simulink model "baseModel"  (R2016b)
settings: Solver=ode14x  StartTime=0.0  StopTime=20  FixedStep=0.01  RelTol=1e-3
values from neighbouring files (symbols this model uses):
  b = (Km*Kb/R)*((2*pi/60))^2    (= 2.64985465309e-07)    [params.m]
  encRes = 64    [params.m]
  gearRatio = 4096/27    (= 151.703703704)    [params.m]
  geom_factor = (0.160 + 0.146)/2    (= 0.153)    [params.m]
  J = 2.7*(10^(-7))    (= 2.7e-07)    [params.m]
  Kb = 0.00152/(2*pi/60)    (= 0.01451493081)    [params.m]
  Km = 0.0145    [params.m]
  L = 0.0002    [params.m]
  pwmRes = 4096    [params.m]
  R = 8.71    [params.m]
  supplyVoltage = 12    [params.m]
  wheelRadius = 0.03    [params.m]
libraries: simulink x7
settings Model: Creator=Mundt  LastModifiedBy=Mundt

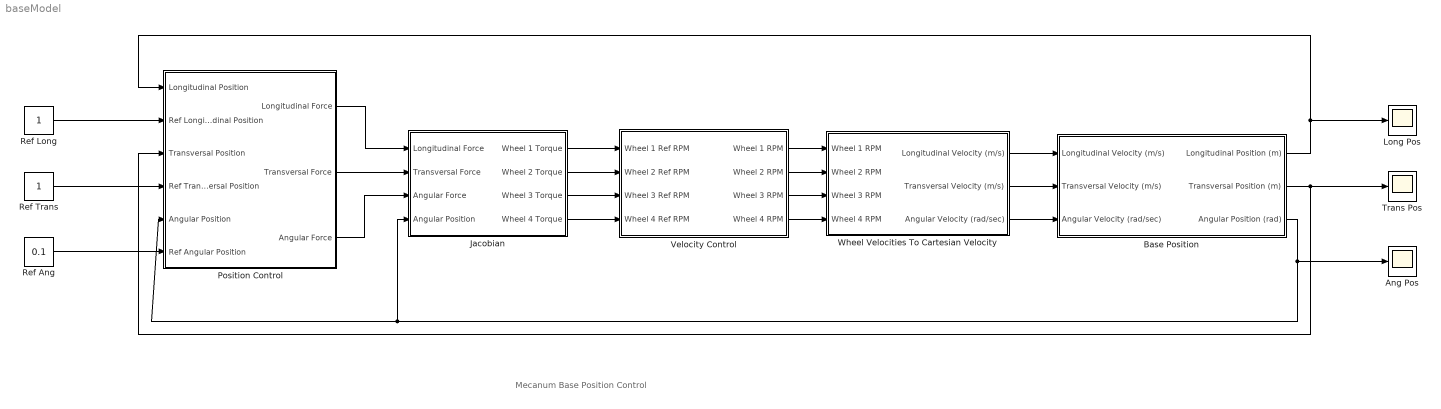
== system baseModel ==
  note: Mecanum Base Position Control
  Ang Pos : Scope
  Base Position : Subsystem
  Jacobian : Subsystem
  Long Pos : Scope
  Position Control : Subsystem
  Ref Ang : Constant  Value=0.1
  Ref Long : Constant
  Ref Trans : Constant
  Trans Pos : Scope
  Velocity Control : Subsystem
  Wheel Velocities To Cartesian Velocity : Subsystem
  wires:
  Velocity Control/1(Wheel 1 RPM) -> Wheel Velocities To Cartesian Velocity/1(Wheel 1 RPM)
  Velocity Control/2(Wheel 2 RPM) -> Wheel Velocities To Cartesian Velocity/2(Wheel 2 RPM)
  Velocity Control/3(Wheel 3 RPM) -> Wheel Velocities To Cartesian Velocity/3(Wheel 3 RPM)
  Velocity Control/4(Wheel 4 RPM) -> Wheel Velocities To Cartesian Velocity/4(Wheel 4 RPM)
  Jacobian/1(Wheel 1 Torque) -> Velocity Control/1(Wheel 1 Ref RPM)
  Jacobian/2(Wheel 2 Torque) -> Velocity Control/2(Wheel 2 Ref RPM)
  Jacobian/3(Wheel 3 Torque) -> Velocity Control/3(Wheel 3 Ref RPM)
  Jacobian/4(Wheel 4 Torque) -> Velocity Control/4(Wheel 4 Ref RPM)
  Wheel Velocities To Cartesian Velocity/1(Longitudinal Velocity (m/s)) -> Base Position/1(Longitudinal Velocity (m/s))
  Wheel Velocities To Cartesian Velocity/2(Transversal Velocity (m/s)) -> Base Position/2(Transversal Velocity (m/s))
  Wheel Velocities To Cartesian Velocity/3(Angular Velocity (rad/sec)) -> Base Position/3(Angular Velocity (rad/sec))
  Base Position/3(Angular Position (rad)) -> Ang Pos/1, Position Control/5(Angular Position), Jacobian/4(Angular Position)
  Position Control/1(Longitudinal Force) -> Jacobian/1(Longitudinal Force)
  Position Control/2(Transversal Force) -> Jacobian/2(Transversal Force)
  Position Control/3(Angular Force) -> Jacobian/3(Angular Force)
  Base Position/1(Longitudinal Position (m)) -> Long Pos/1, Position Control/1(Longitudinal Position)
  Ref Long/1 -> Position Control/2(Ref Longitudinal Position)
  Base Position/2(Transversal Position (m)) -> Trans Pos/1, Position Control/3(Transversal Position)
  Ref Trans/1 -> Position Control/4(Ref Transversal Position)
  Ref Ang/1 -> Position Control/6(Ref Angular Position)

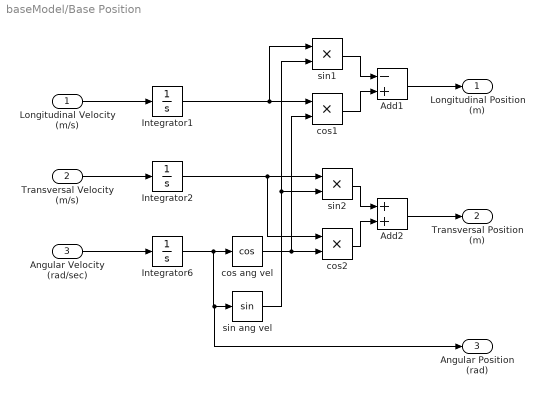
== system baseModel/Base Position ==
  Longitudinal Velocity (m/s) : Inport
  Transversal Velocity (m/s) : Inport  Port=2
  Angular Velocity (rad/sec) : Inport  Port=3
  Add1 : Sum  Inputs=-+
  Add2 : Sum
  Integrator1 : Integrator
  Integrator2 : Integrator
  Integrator6 : Integrator
  cos ang vel : Trigonometry  Operator=cos
  cos1 : Product
  cos2 : Product
  sin ang vel : Trigonometry
  sin1 : Product
  sin2 : Product
  Longitudinal Position (m) : Outport
  Transversal Position (m) : Outport  Port=2
  Angular Position (rad) : Outport  Port=3
  wires:
  Angular Velocity (rad/sec)/1 -> Integrator6/1
  Longitudinal Velocity (m/s)/1 -> Integrator1/1
  Transversal Velocity (m/s)/1 -> Integrator2/1
  Integrator6/1 -> Angular Position (rad)/1, sin ang vel/1, cos ang vel/1
  Integrator2/1 -> cos2/1, sin2/1
  Integrator1/1 -> sin1/1, cos1/1
  cos ang vel/1 -> cos1/2, cos2/2
  sin ang vel/1 -> sin2/2, sin1/2
  cos1/1 -> Add1/2
  sin1/1 -> Add1/1
  Add1/1 -> Longitudinal Position (m)/1
  sin2/1 -> Add2/1
  cos2/1 -> Add2/2
  Add2/1 -> Transversal Position (m)/1

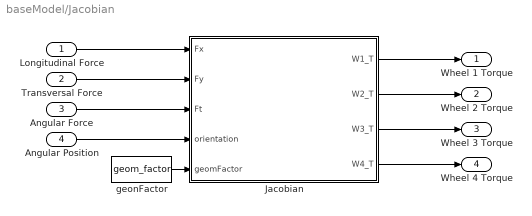
== system baseModel/Jacobian ==
  Longitudinal Force : Inport
  Transversal Force : Inport  Port=2
  Angular Force : Inport  Port=3
  Angular Position : Inport  Port=4
  Jacobian : MATLAB Function  TreatAsAtomicUnit=on
  geonFactor : Constant  Value=geom_factor
  Wheel 1 Torque : Outport
  Wheel 2 Torque : Outport  Port=2
  Wheel 3 Torque : Outport  Port=3
  Wheel 4 Torque : Outport  Port=4
  wires:
  Jacobian/2(W2_T) -> Wheel 2 Torque/1
  Jacobian/1(W1_T) -> Wheel 1 Torque/1
  Jacobian/3(W3_T) -> Wheel 3 Torque/1
  Jacobian/4(W4_T) -> Wheel 4 Torque/1
  Transversal Force/1 -> Jacobian/2(Fy)
  Angular Force/1 -> Jacobian/3(Ft)
  Angular Position/1 -> Jacobian/4(orientation)
  Longitudinal Force/1 -> Jacobian/1(Fx)
  geonFactor/1 -> Jacobian/5(geomFactor)

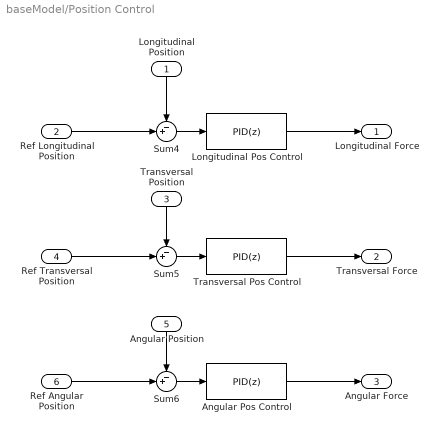
== system baseModel/Position Control ==
  Longitudinal Position : Inport
  Ref Longitudinal Position : Inport  Port=2
  Transversal Position : Inport  Port=3
  Ref Transversal Position : Inport  Port=4
  Angular Position : Inport  Port=5
  Ref Angular Position : Inport  Port=6
  Angular Pos Control : simulink/Continuous/PID Controller  Controller=PID  TimeDomain=Discrete-time  SampleTime=0.1  IntegratorMethod=Forward Euler  FilterMethod=Forward Euler  Form=Parallel  UseFilter=off  ControllerParametersSource=internal  P=1000  I=0  D=0  N=2.61986386907553  InitialConditionSource=internal  InitialConditionForIntegrator=0  InitialConditionForFilter=0  ExternalReset=none  LimitOutput=on  UpperSaturationLimit=4096  LowerSaturationLimit=-4096  LinearizeAsGain=off  AntiWindupMode=none  Kb=1  TrackingMode=off  Kt=1  PParamMin=[]  PParamMax=[]  IParamMin=[]  IParamMax=[]  DParamMin=[]  DParamMax=[]  NParamMin=[]  NParamMax=[]  KbParamMin=[]  KbParamMax=[]  KtParamMin=[]  KtParamMax=[]  POutMin=[]  POutMax=[]  IOutMin=[]  IOutMax=[]  DOutMin=[]  DOutMax=[]  NOutMin=[]  NOutMax=[]  KbOutMin=[]  KbOutMax=[]  KtOutMin=[]  KtOutMax=[]  IntegratorOutMin=[]  IntegratorOutMax=[]  FilterOutMin=[]  FilterOutMax=[]  SumOutMin=[]  SumOutMax=[]  SumI1OutMin=[]  SumI1OutMax=[]  SumI2OutMin=[]  SumI2OutMax=[]  SumI3OutMin=[]  SumI3OutMax=[]  SumDOutMin=[]  SumDOutMax=[]  SaturationOutMin=[]  SaturationOutMax=[]  IntegratorContinuousStateAttributes=''  IntegratorStateMustResolveToSignalObject=off  IntegratorRTWStateStorageClass=Auto  FilterContinuousStateAttributes=''  FilterStateMustResolveToSignalObject=off  FilterRTWStateStorageClass=Auto  DifferentiatorICPrevScaledInput=0  DifferentiatorOutMin=[]  DifferentiatorOutMax=[]
  Longitudinal Pos Control : simulink/Continuous/PID Controller  Controller=PID  TimeDomain=Discrete-time  SampleTime=0.1  IntegratorMethod=Forward Euler  FilterMethod=Forward Euler  Form=Parallel  UseFilter=off  ControllerParametersSource=internal  P=2000  I=0  D=0  N=2.61986386907553  InitialConditionSource=internal  InitialConditionForIntegrator=0  InitialConditionForFilter=0  ExternalReset=none  LimitOutput=on  UpperSaturationLimit=4096  LowerSaturationLimit=-4096  LinearizeAsGain=off  AntiWindupMode=none  Kb=1  TrackingMode=off  Kt=1  PParamMin=[]  PParamMax=[]  IParamMin=[]  IParamMax=[]  DParamMin=[]  DParamMax=[]  NParamMin=[]  NParamMax=[]  KbParamMin=[]  KbParamMax=[]  KtParamMin=[]  KtParamMax=[]  POutMin=[]  POutMax=[]  IOutMin=[]  IOutMax=[]  DOutMin=[]  DOutMax=[]  NOutMin=[]  NOutMax=[]  KbOutMin=[]  KbOutMax=[]  KtOutMin=[]  KtOutMax=[]  IntegratorOutMin=[]  IntegratorOutMax=[]  FilterOutMin=[]  FilterOutMax=[]  SumOutMin=[]  SumOutMax=[]  SumI1OutMin=[]  SumI1OutMax=[]  SumI2OutMin=[]  SumI2OutMax=[]  SumI3OutMin=[]  SumI3OutMax=[]  SumDOutMin=[]  SumDOutMax=[]  SaturationOutMin=[]  SaturationOutMax=[]  IntegratorContinuousStateAttributes=''  IntegratorStateMustResolveToSignalObject=off  IntegratorRTWStateStorageClass=Auto  FilterContinuousStateAttributes=''  FilterStateMustResolveToSignalObject=off  FilterRTWStateStorageClass=Auto  DifferentiatorICPrevScaledInput=0  DifferentiatorOutMin=[]  DifferentiatorOutMax=[]
  Sum4 : Sum  Inputs=-+|
  Sum5 : Sum  Inputs=-+|
  Sum6 : Sum  Inputs=-+|
  Transversal Pos Control : simulink/Continuous/PID Controller  Controller=PID  TimeDomain=Discrete-time  SampleTime=0.1  IntegratorMethod=Forward Euler  FilterMethod=Forward Euler  Form=Parallel  UseFilter=off  ControllerParametersSource=internal  P=2000  I=0  D=0  N=2.61986386907553  InitialConditionSource=internal  InitialConditionForIntegrator=0  InitialConditionForFilter=0  ExternalReset=none  LimitOutput=on  UpperSaturationLimit=4096  LowerSaturationLimit=-4096  LinearizeAsGain=off  AntiWindupMode=none  Kb=1  TrackingMode=off  Kt=1  PParamMin=[]  PParamMax=[]  IParamMin=[]  IParamMax=[]  DParamMin=[]  DParamMax=[]  NParamMin=[]  NParamMax=[]  KbParamMin=[]  KbParamMax=[]  KtParamMin=[]  KtParamMax=[]  POutMin=[]  POutMax=[]  IOutMin=[]  IOutMax=[]  DOutMin=[]  DOutMax=[]  NOutMin=[]  NOutMax=[]  KbOutMin=[]  KbOutMax=[]  KtOutMin=[]  KtOutMax=[]  IntegratorOutMin=[]  IntegratorOutMax=[]  FilterOutMin=[]  FilterOutMax=[]  SumOutMin=[]  SumOutMax=[]  SumI1OutMin=[]  SumI1OutMax=[]  SumI2OutMin=[]  SumI2OutMax=[]  SumI3OutMin=[]  SumI3OutMax=[]  SumDOutMin=[]  SumDOutMax=[]  SaturationOutMin=[]  SaturationOutMax=[]  IntegratorContinuousStateAttributes=''  IntegratorStateMustResolveToSignalObject=off  IntegratorRTWStateStorageClass=Auto  FilterContinuousStateAttributes=''  FilterStateMustResolveToSignalObject=off  FilterRTWStateStorageClass=Auto  DifferentiatorICPrevScaledInput=0  DifferentiatorOutMin=[]  DifferentiatorOutMax=[]
  Longitudinal Force : Outport
  Transversal Force : Outport  Port=2
  Angular Force : Outport  Port=3
  wires:
  Angular Position/1 -> Sum6/1
  Longitudinal Position/1 -> Sum4/1
  Angular Pos Control/1 -> Angular Force/1
  Transversal Pos Control/1 -> Transversal Force/1
  Transversal Position/1 -> Sum5/1
  Sum4/1 -> Longitudinal Pos Control/1
  Ref Angular Position/1 -> Sum6/2
  Sum5/1 -> Transversal Pos Control/1
  Ref Transversal Position/1 -> Sum5/2
  Sum6/1 -> Angular Pos Control/1
  Ref Longitudinal Position/1 -> Sum4/2
  Longitudinal Pos Control/1 -> Longitudinal Force/1

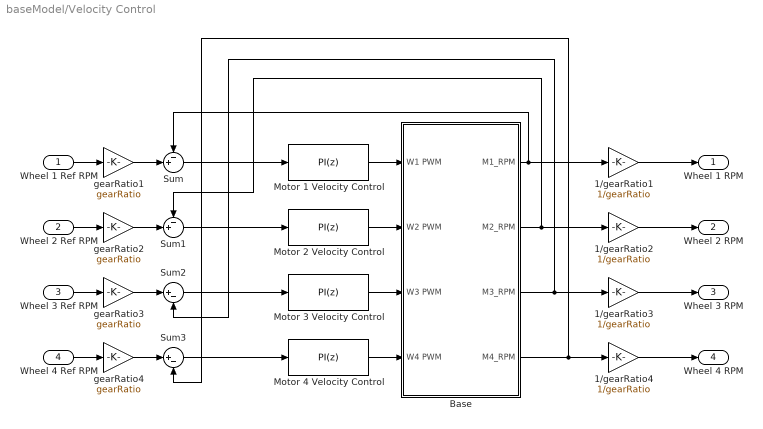
== system baseModel/Velocity Control ==
  Wheel 1 Ref RPM : Inport
  Wheel 2 Ref RPM : Inport  Port=2
  Wheel 3 Ref RPM : Inport  Port=3
  Wheel 4 Ref RPM : Inport  Port=4
  1/gearRatio{1..4} (4 alike) : Gain  Gain=1/gearRatio
  Base : Subsystem
  Motor 1 Velocity Control : simulink/Continuous/PID Controller  Controller=PI  TimeDomain=Discrete-time  SampleTime=0.01  IntegratorMethod=Forward Euler  FilterMethod=Forward Euler  Form=Parallel  UseFilter=on  ControllerParametersSource=internal  P=0.39976  I=23.7406  D=0  N=100  InitialConditionSource=internal  InitialConditionForIntegrator=0  InitialConditionForFilter=0  ExternalReset=none  LimitOutput=off  UpperSaturationLimit=inf  LowerSaturationLimit=-inf  LinearizeAsGain=off  AntiWindupMode=none  Kb=1  TrackingMode=off  Kt=1  PParamMin=[]  PParamMax=[]  IParamMin=[]  IParamMax=[]  DParamMin=[]  DParamMax=[]  NParamMin=[]  NParamMax=[]  KbParamMin=[]  KbParamMax=[]  KtParamMin=[]  KtParamMax=[]  POutMin=[]  POutMax=[]  IOutMin=[]  IOutMax=[]  DOutMin=[]  DOutMax=[]  NOutMin=[]  NOutMax=[]  KbOutMin=[]  KbOutMax=[]  KtOutMin=[]  KtOutMax=[]  IntegratorOutMin=[]  IntegratorOutMax=[]  FilterOutMin=[]  FilterOutMax=[]  SumOutMin=[]  SumOutMax=[]  SumI1OutMin=[]  SumI1OutMax=[]  SumI2OutMin=[]  SumI2OutMax=[]  SumI3OutMin=[]  SumI3OutMax=[]  SumDOutMin=[]  SumDOutMax=[]  SaturationOutMin=[]  SaturationOutMax=[]  IntegratorContinuousStateAttributes=''  IntegratorStateMustResolveToSignalObject=off  IntegratorRTWStateStorageClass=Auto  FilterContinuousStateAttributes=''  FilterStateMustResolveToSignalObject=off  FilterRTWStateStorageClass=Auto  DifferentiatorICPrevScaledInput=0  DifferentiatorOutMin=[]  DifferentiatorOutMax=[]
  Motor 2 Velocity Control : simulink/Continuous/PID Controller  Controller=PI  TimeDomain=Discrete-time  SampleTime=0.01  IntegratorMethod=Forward Euler  FilterMethod=Forward Euler  Form=Parallel  UseFilter=on  ControllerParametersSource=internal  P=0.39976  I=23.7406  D=0  N=100  InitialConditionSource=internal  InitialConditionForIntegrator=0  InitialConditionForFilter=0  ExternalReset=none  LimitOutput=off  UpperSaturationLimit=inf  LowerSaturationLimit=-inf  LinearizeAsGain=off  AntiWindupMode=none  Kb=1  TrackingMode=off  Kt=1  PParamMin=[]  PParamMax=[]  IParamMin=[]  IParamMax=[]  DParamMin=[]  DParamMax=[]  NParamMin=[]  NParamMax=[]  KbParamMin=[]  KbParamMax=[]  KtParamMin=[]  KtParamMax=[]  POutMin=[]  POutMax=[]  IOutMin=[]  IOutMax=[]  DOutMin=[]  DOutMax=[]  NOutMin=[]  NOutMax=[]  KbOutMin=[]  KbOutMax=[]  KtOutMin=[]  KtOutMax=[]  IntegratorOutMin=[]  IntegratorOutMax=[]  FilterOutMin=[]  FilterOutMax=[]  SumOutMin=[]  SumOutMax=[]  SumI1OutMin=[]  SumI1OutMax=[]  SumI2OutMin=[]  SumI2OutMax=[]  SumI3OutMin=[]  SumI3OutMax=[]  SumDOutMin=[]  SumDOutMax=[]  SaturationOutMin=[]  SaturationOutMax=[]  IntegratorContinuousStateAttributes=''  IntegratorStateMustResolveToSignalObject=off  IntegratorRTWStateStorageClass=Auto  FilterContinuousStateAttributes=''  FilterStateMustResolveToSignalObject=off  FilterRTWStateStorageClass=Auto  DifferentiatorICPrevScaledInput=0  DifferentiatorOutMin=[]  DifferentiatorOutMax=[]
  Motor 3 Velocity Control : simulink/Continuous/PID Controller  Controller=PI  TimeDomain=Discrete-time  SampleTime=0.01  IntegratorMethod=Forward Euler  FilterMethod=Forward Euler  Form=Parallel  UseFilter=on  ControllerParametersSource=internal  P=0.39976  I=23.7406  D=0  N=100  InitialConditionSource=internal  InitialConditionForIntegrator=0  InitialConditionForFilter=0  ExternalReset=none  LimitOutput=off  UpperSaturationLimit=inf  LowerSaturationLimit=-inf  LinearizeAsGain=off  AntiWindupMode=none  Kb=1  TrackingMode=off  Kt=1  PParamMin=[]  PParamMax=[]  IParamMin=[]  IParamMax=[]  DParamMin=[]  DParamMax=[]  NParamMin=[]  NParamMax=[]  KbParamMin=[]  KbParamMax=[]  KtParamMin=[]  KtParamMax=[]  POutMin=[]  POutMax=[]  IOutMin=[]  IOutMax=[]  DOutMin=[]  DOutMax=[]  NOutMin=[]  NOutMax=[]  KbOutMin=[]  KbOutMax=[]  KtOutMin=[]  KtOutMax=[]  IntegratorOutMin=[]  IntegratorOutMax=[]  FilterOutMin=[]  FilterOutMax=[]  SumOutMin=[]  SumOutMax=[]  SumI1OutMin=[]  SumI1OutMax=[]  SumI2OutMin=[]  SumI2OutMax=[]  SumI3OutMin=[]  SumI3OutMax=[]  SumDOutMin=[]  SumDOutMax=[]  SaturationOutMin=[]  SaturationOutMax=[]  IntegratorContinuousStateAttributes=''  IntegratorStateMustResolveToSignalObject=off  IntegratorRTWStateStorageClass=Auto  FilterContinuousStateAttributes=''  FilterStateMustResolveToSignalObject=off  FilterRTWStateStorageClass=Auto  DifferentiatorICPrevScaledInput=0  DifferentiatorOutMin=[]  DifferentiatorOutMax=[]
  Motor 4 Velocity Control : simulink/Continuous/PID Controller  Controller=PI  TimeDomain=Discrete-time  SampleTime=0.01  IntegratorMethod=Forward Euler  FilterMethod=Forward Euler  Form=Parallel  UseFilter=on  ControllerParametersSource=internal  P=0.39976  I=23.7406  D=0  N=100  InitialConditionSource=internal  InitialConditionForIntegrator=0  InitialConditionForFilter=0  ExternalReset=none  LimitOutput=off  UpperSaturationLimit=inf  LowerSaturationLimit=-inf  LinearizeAsGain=off  AntiWindupMode=none  Kb=1  TrackingMode=off  Kt=1  PParamMin=[]  PParamMax=[]  IParamMin=[]  IParamMax=[]  DParamMin=[]  DParamMax=[]  NParamMin=[]  NParamMax=[]  KbParamMin=[]  KbParamMax=[]  KtParamMin=[]  KtParamMax=[]  POutMin=[]  POutMax=[]  IOutMin=[]  IOutMax=[]  DOutMin=[]  DOutMax=[]  NOutMin=[]  NOutMax=[]  KbOutMin=[]  KbOutMax=[]  KtOutMin=[]  KtOutMax=[]  IntegratorOutMin=[]  IntegratorOutMax=[]  FilterOutMin=[]  FilterOutMax=[]  SumOutMin=[]  SumOutMax=[]  SumI1OutMin=[]  SumI1OutMax=[]  SumI2OutMin=[]  SumI2OutMax=[]  SumI3OutMin=[]  SumI3OutMax=[]  SumDOutMin=[]  SumDOutMax=[]  SaturationOutMin=[]  SaturationOutMax=[]  IntegratorContinuousStateAttributes=''  IntegratorStateMustResolveToSignalObject=off  IntegratorRTWStateStorageClass=Auto  FilterContinuousStateAttributes=''  FilterStateMustResolveToSignalObject=off  FilterRTWStateStorageClass=Auto  DifferentiatorICPrevScaledInput=0  DifferentiatorOutMin=[]  DifferentiatorOutMax=[]
  Sum : Sum  Inputs=-+|
  Sum1 : Sum  Inputs=-+|
  Sum2 : Sum  Inputs=|+-
  Sum3 : Sum  Inputs=|+-
  gearRatio1 : Gain  Gain=gearRatio
  gearRatio2 : Gain  Gain=gearRatio
  gearRatio3 : Gain  Gain=gearRatio
  "gearRatio4 " : Gain  Gain=gearRatio
  Wheel 1 RPM : Outport
  Wheel 2 RPM : Outport  Port=2
  Wheel 3 RPM : Outport  Port=3
  Wheel 4 RPM : Outport  Port=4
  wires:
  Wheel 4 Ref RPM/1 -> "gearRatio4 "/1
  Wheel 3 Ref RPM/1 -> gearRatio3/1
  gearRatio2/1 -> Sum1/2
  Sum/1 -> Motor 1 Velocity Control/1
  Wheel 1 Ref RPM/1 -> gearRatio1/1
  "gearRatio4 "/1 -> Sum3/1
  Wheel 2 Ref RPM/1 -> gearRatio2/1
  Base/1(M1_RPM) -> Sum/1, 1/gearRatio1/1
  Base/2(M2_RPM) -> Sum1/1, 1/gearRatio2/1
  Sum3/1 -> Motor 4 Velocity Control/1
  Base/3(M3_RPM) -> Sum2/2, 1/gearRatio3/1
  Sum1/1 -> Motor 2 Velocity Control/1
  Sum2/1 -> Motor 3 Velocity Control/1
  Base/4(M4_RPM) -> Sum3/2, 1/gearRatio4/1
  Motor 1 Velocity Control/1 -> Base/1(W1 PWM)
  Motor 2 Velocity Control/1 -> Base/2(W2 PWM)
  Motor 3 Velocity Control/1 -> Base/3(W3 PWM)
  Motor 4 Velocity Control/1 -> Base/4(W4 PWM)
  gearRatio1/1 -> Sum/2
  gearRatio3/1 -> Sum2/1
  1/gearRatio1/1 -> Wheel 1 RPM/1
  1/gearRatio2/1 -> Wheel 2 RPM/1
  1/gearRatio3/1 -> Wheel 3 RPM/1
  1/gearRatio4/1 -> Wheel 4 RPM/1

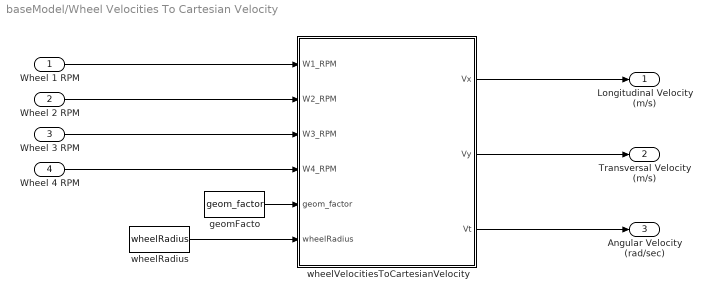
== system baseModel/Wheel Velocities To Cartesian Velocity ==
  Wheel 1 RPM : Inport
  Wheel 2 RPM : Inport  Port=2
  Wheel 3 RPM : Inport  Port=3
  Wheel 4 RPM : Inport  Port=4
  geomFacto : Constant  Value=geom_factor
  wheelRadius : Constant  Value=wheelRadius
  wheelVelocitiesToCartesianVelocity : MATLAB Function  TreatAsAtomicUnit=on
  Longitudinal Velocity (m/s) : Outport
  Transversal Velocity (m/s) : Outport  Port=2
  Angular Velocity (rad/sec) : Outport  Port=3
  wires:
  wheelRadius/1 -> wheelVelocitiesToCartesianVelocity/6(wheelRadius)
  Wheel 2 RPM/1 -> wheelVelocitiesToCartesianVelocity/2(W2_RPM)
  Wheel 4 RPM/1 -> wheelVelocitiesToCartesianVelocity/4(W4_RPM)
  geomFacto/1 -> wheelVelocitiesToCartesianVelocity/5(geom_factor)
  Wheel 1 RPM/1 -> wheelVelocitiesToCartesianVelocity/1(W1_RPM)
  Wheel 3 RPM/1 -> wheelVelocitiesToCartesianVelocity/3(W3_RPM)
  wheelVelocitiesToCartesianVelocity/3(Vt) -> Angular Velocity (rad/sec)/1
  wheelVelocitiesToCartesianVelocity/1(Vx) -> Longitudinal Velocity (m/s)/1
  wheelVelocitiesToCartesianVelocity/2(Vy) -> Transversal Velocity (m/s)/1

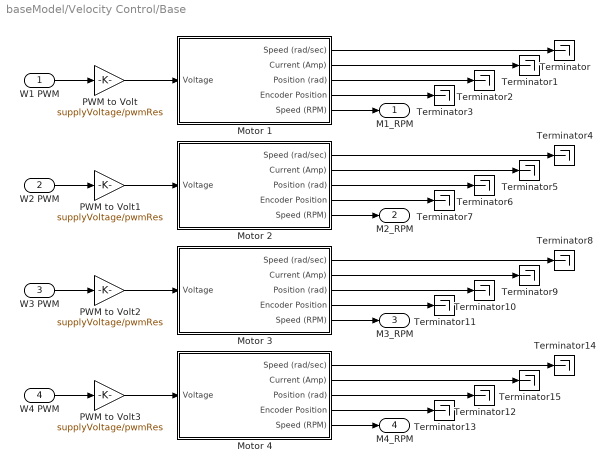
== system baseModel/Velocity Control/Base ==
  W1 PWM : Inport
  W2 PWM : Inport  Port=2
  W3 PWM : Inport  Port=3
  W4 PWM : Inport  Port=4
  Motor 1 : Subsystem
  Motor 2 : Subsystem
  Motor 3 : Subsystem
  Motor 4 : Subsystem
  PWM to Volt{,1..3} (4 alike) : Gain  Gain=supplyVoltage/pwmRes
  Terminator{,1..15} (16 alike) : Terminator
  M1_RPM : Outport
  M2_RPM : Outport  Port=2
  M3_RPM : Outport  Port=3
  M4_RPM : Outport  Port=4
  wires:
  W1 PWM/1 -> PWM to Volt/1
  PWM to Volt/1 -> Motor 1/1(Voltage)
  PWM to Volt1/1 -> Motor 2/1(Voltage)
  W2 PWM/1 -> PWM to Volt1/1
  PWM to Volt2/1 -> Motor 3/1(Voltage)
  W3 PWM/1 -> PWM to Volt2/1
  PWM to Volt3/1 -> Motor 4/1(Voltage)
  W4 PWM/1 -> PWM to Volt3/1
  Motor 1/5(Speed (RPM)) -> M1_RPM/1
  Motor 2/5(Speed (RPM)) -> M2_RPM/1
  Motor 3/5(Speed (RPM)) -> M3_RPM/1
  Motor 4/5(Speed (RPM)) -> M4_RPM/1
  Motor 1/1(Speed (rad/sec)) -> Terminator/1
  Motor 1/2(Current (Amp)) -> Terminator1/1
  Motor 1/3(Position (rad)) -> Terminator2/1
  Motor 1/4(Encoder Position) -> Terminator3/1
  Motor 2/1(Speed (rad/sec)) -> Terminator4/1
  Motor 2/2(Current (Amp)) -> Terminator5/1
  Motor 2/3(Position (rad)) -> Terminator6/1
  Motor 2/4(Encoder Position) -> Terminator7/1
  Motor 3/1(Speed (rad/sec)) -> Terminator8/1
  Motor 3/2(Current (Amp)) -> Terminator9/1
  Motor 3/3(Position (rad)) -> Terminator10/1
  Motor 3/4(Encoder Position) -> Terminator11/1
  Motor 4/1(Speed (rad/sec)) -> Terminator14/1
  Motor 4/2(Current (Amp)) -> Terminator15/1
  Motor 4/3(Position (rad)) -> Terminator12/1
  Motor 4/4(Encoder Position) -> Terminator13/1

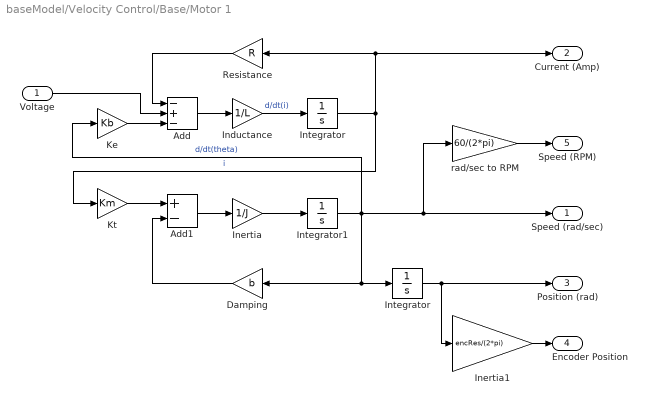
== system baseModel/Velocity Control/Base/Motor 1 ==
  Voltage : Inport
  Add : Sum  Inputs=-+-
  Add1 : Sum  Inputs=+-
  Damping : Gain  Gain=b
  Inductance : Gain  Gain=1/L
  Inertia : Gain  Gain=1/J
  Inertia1 : Gain  Gain=encRes/(2*pi)
  Integrator : Integrator
  "Integrator " : Integrator
  Integrator1 : Integrator
  Ke : Gain  Gain=Kb
  Kt : Gain  Gain=Km
  Resistance : Gain  Gain=R
  rad/sec to RPM : Gain  Gain=60/(2*pi)
  Speed (rad/sec) : Outport
  Current (Amp) : Outport  Port=2
  Position (rad) : Outport  Port=3
  Encoder Position : Outport  Port=4
  Speed (RPM) : Outport  Port=5
  wires:
  Resistance/1 -> Add/1
  Ke/1 -> Add/3
  Inertia/1 -> Integrator1/1
  Voltage/1 -> Add/2
  Damping/1 -> Add1/2
  Kt/1 -> Add1/1
  Add1/1 -> Inertia/1
  Inductance/1 -> Integrator/1  "d/dt(i)"
  Add/1 -> Inductance/1
  Integrator1/1 -> rad/sec to RPM/1, Speed (rad/sec)/1, Ke/1, "Integrator "/1, Damping/1  "d/dt(theta)"
  Integrator/1 -> Current (Amp)/1, Resistance/1, Kt/1  "i"
  "Integrator "/1 -> Inertia1/1, Position (rad)/1
  Inertia1/1 -> Encoder Position/1
  rad/sec to RPM/1 -> Speed (RPM)/1

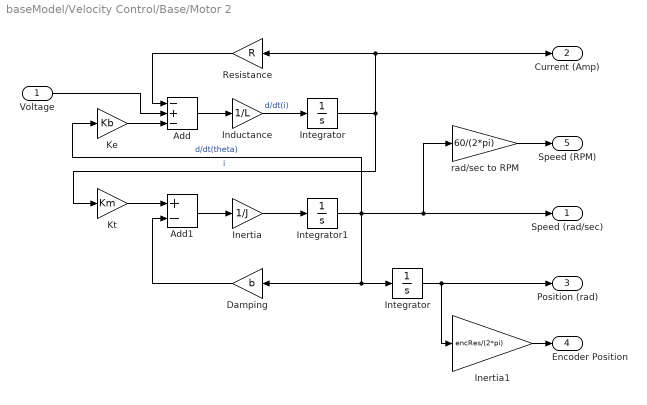
== system baseModel/Velocity Control/Base/Motor 2 ==
  Voltage : Inport
  Add : Sum  Inputs=-+-
  Add1 : Sum  Inputs=+-
  Damping : Gain  Gain=b
  Inductance : Gain  Gain=1/L
  Inertia : Gain  Gain=1/J
  Inertia1 : Gain  Gain=encRes/(2*pi)
  Integrator : Integrator
  "Integrator " : Integrator
  Integrator1 : Integrator
  Ke : Gain  Gain=Kb
  Kt : Gain  Gain=Km
  Resistance : Gain  Gain=R
  rad/sec to RPM : Gain  Gain=60/(2*pi)
  Speed (rad/sec) : Outport
  Current (Amp) : Outport  Port=2
  Position (rad) : Outport  Port=3
  Encoder Position : Outport  Port=4
  Speed (RPM) : Outport  Port=5
  wires:
  rad/sec to RPM/1 -> Speed (RPM)/1
  Inertia1/1 -> Encoder Position/1
  "Integrator "/1 -> Position (rad)/1, Inertia1/1
  Integrator/1 -> Kt/1, Resistance/1, Current (Amp)/1  "i"
  Integrator1/1 -> Damping/1, "Integrator "/1, Ke/1, Speed (rad/sec)/1, rad/sec to RPM/1  "d/dt(theta)"
  Add/1 -> Inductance/1
  Inductance/1 -> Integrator/1  "d/dt(i)"
  Add1/1 -> Inertia/1
  Kt/1 -> Add1/1
  Damping/1 -> Add1/2
  Voltage/1 -> Add/2
  Inertia/1 -> Integrator1/1
  Ke/1 -> Add/3
  Resistance/1 -> Add/1

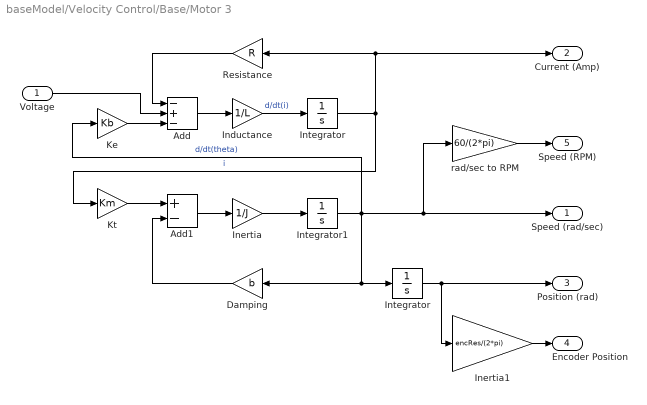
== system baseModel/Velocity Control/Base/Motor 3 ==
  Voltage : Inport
  Add : Sum  Inputs=-+-
  Add1 : Sum  Inputs=+-
  Damping : Gain  Gain=b
  Inductance : Gain  Gain=1/L
  Inertia : Gain  Gain=1/J
  Inertia1 : Gain  Gain=encRes/(2*pi)
  Integrator : Integrator
  "Integrator " : Integrator
  Integrator1 : Integrator
  Ke : Gain  Gain=Kb
  Kt : Gain  Gain=Km
  Resistance : Gain  Gain=R
  rad/sec to RPM : Gain  Gain=60/(2*pi)
  Speed (rad/sec) : Outport
  Current (Amp) : Outport  Port=2
  Position (rad) : Outport  Port=3
  Encoder Position : Outport  Port=4
  Speed (RPM) : Outport  Port=5
  wires:
  rad/sec to RPM/1 -> Speed (RPM)/1
  Inertia1/1 -> Encoder Position/1
  "Integrator "/1 -> Position (rad)/1, Inertia1/1
  Integrator/1 -> Kt/1, Resistance/1, Current (Amp)/1  "i"
  Integrator1/1 -> Damping/1, "Integrator "/1, Ke/1, Speed (rad/sec)/1, rad/sec to RPM/1  "d/dt(theta)"
  Add/1 -> Inductance/1
  Inductance/1 -> Integrator/1  "d/dt(i)"
  Add1/1 -> Inertia/1
  Kt/1 -> Add1/1
  Damping/1 -> Add1/2
  Voltage/1 -> Add/2
  Inertia/1 -> Integrator1/1
  Ke/1 -> Add/3
  Resistance/1 -> Add/1

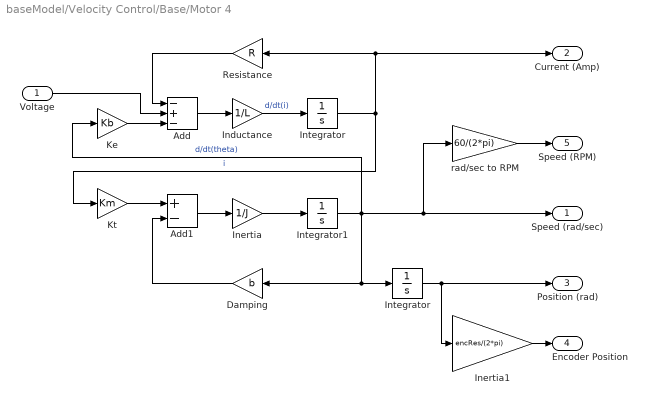
== system baseModel/Velocity Control/Base/Motor 4 ==
  Voltage : Inport
  Add : Sum  Inputs=-+-
  Add1 : Sum  Inputs=+-
  Damping : Gain  Gain=b
  Inductance : Gain  Gain=1/L
  Inertia : Gain  Gain=1/J
  Inertia1 : Gain  Gain=encRes/(2*pi)
  Integrator : Integrator
  "Integrator " : Integrator
  Integrator1 : Integrator
  Ke : Gain  Gain=Kb
  Kt : Gain  Gain=Km
  Resistance : Gain  Gain=R
  rad/sec to RPM : Gain  Gain=60/(2*pi)
  Speed (rad/sec) : Outport
  Current (Amp) : Outport  Port=2
  Position (rad) : Outport  Port=3
  Encoder Position : Outport  Port=4
  Speed (RPM) : Outport  Port=5
  wires:
  Resistance/1 -> Add/1
  Ke/1 -> Add/3
  Inertia/1 -> Integrator1/1
  Voltage/1 -> Add/2
  Damping/1 -> Add1/2
  Kt/1 -> Add1/1
  Add1/1 -> Inertia/1
  Inductance/1 -> Integrator/1  "d/dt(i)"
  Add/1 -> Inductance/1
  Integrator1/1 -> rad/sec to RPM/1, Speed (rad/sec)/1, Ke/1, "Integrator "/1, Damping/1  "d/dt(theta)"
  Integrator/1 -> Current (Amp)/1, Resistance/1, Kt/1  "i"
  "Integrator "/1 -> Inertia1/1, Position (rad)/1
  Inertia1/1 -> Encoder Position/1
  rad/sec to RPM/1 -> Speed (RPM)/1

== matlab function baseModel/Wheel Velocities To Cartesian Velocity/wheelVelocitiesToCartesianVelocity ==
  data: W1_RPM input; Vx output; W2_RPM input; W3_RPM input; W4_RPM input; Vy output; Vt output; geom_factor input; wheelRadius input
function [Vx, Vy, Vt] = fcn(W1_RPM, W2_RPM, W3_RPM, W4_RPM, geom_factor, wheelRadius )

W1_angVel = W1_RPM * 2 * pi / 60;
W2_angVel = W2_RPM * 2 * pi / 60;
W3_angVel = W3_RPM * 2 * pi / 60;
W4_angVel = W4_RPM * 2 * pi / 60;

Vx = (W1_angVel + W2_angVel + W3_angVel + W4_angVel) * wheelRadius / 4;
Vy = (W1_angVel - W2_angVel - W3_angVel + W4_angVel) * wheelRadius / 4;
Vt = (W1_angVel - W2_angVel + W3_angVel - W4_angVel) * wheelRadius /(4 * geom_factor);

== matlab function baseModel/Jacobian/Jacobian ==
  data: Fx input; W1_T output; Fy input; Ft input; orientation input; W2_T output; W3_T output; W4_T output; geomFactor input
function [W1_T, W2_T, W3_T, W4_T] = fcn(Fx, Fy, Ft, orientation, geomFactor)

W1_T = Fx*(cos(orientation)-sin(orientation))/sqrt(2) + Fy*(sin(orientation)+cos(orientation))/sqrt(2) + Ft*geomFactor*sqrt(2);
W2_T = Fx*(cos(orientation)+sin(orientation))/sqrt(2) + Fy*(sin(orientation)-cos(orientation))/sqrt(2) - Ft*geomFactor*sqrt(2);
W3_T = Fx*(cos(orientation)+sin(orientation))/sqrt(2) + Fy*(sin(orientation)-cos(orientation))/sqrt(2) + Ft*geomFactor*sqrt(2);
W4_T = Fx*(cos(orientation)-sin(orientation))/sqrt(2) + Fy*(sin(orientation)+cos(orientation))/sqrt(2) - Ft*geomFactor*sqrt(2);
